simulink model "HilBlkFilterDemo"  (Simulink 6.0)
settings: Solver=FixedStepDiscrete  StartTime=0.0  StopTime=127/8000  RelTol=1e-3
StopFcn:
  | HilBlkFilterDemo_script('viewResults')
libraries: dspsrcs4 x2, HilLib x1, dsparch4 x1, dspsigops x1
settings Model: Creator=ckalluri  LastModifiedBy=mnazario
settings DataIOCC: SignalLoggingName=sigsOut
settings OptimizationCC: RollThreshold=2
settings DebuggingCC: CheckExecutionContextPreStartOutputMsg=on  CheckExecutionContextRuntimeOutputMsg=on  SolverPrmCheckMsg=none
settings HardwareCC: TargetUnknown=on
settings SFSimCC: SFSimApplyToAllLibs=on  SFSimBuildMode=Incremental

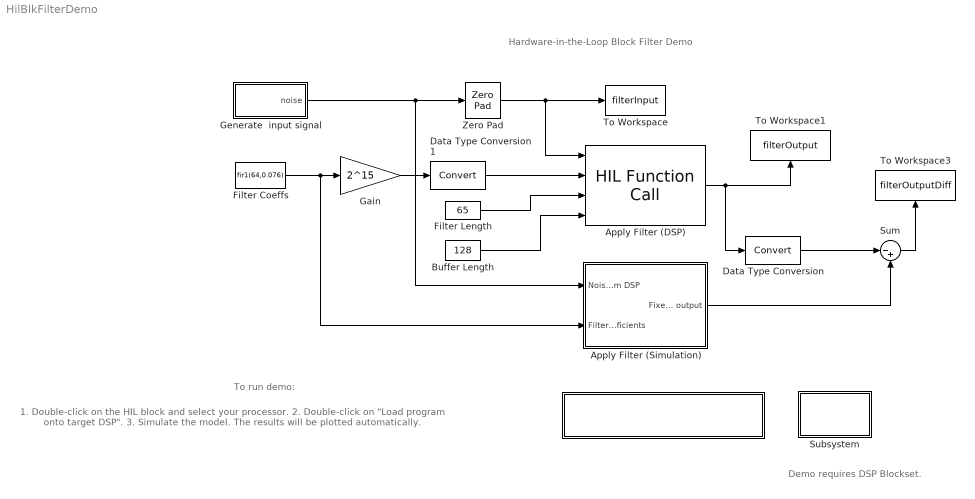
== system HilBlkFilterDemo ==
  note: Hardware-in-the-Loop Block
      | Filter Demo
  note: 1. Double-click on the HIL block and select your processor.
      | 2. Double-click on "Load program onto target DSP".
      | 3. Simulate the model.  The results will be plotted automatically.
  note: Demo requires DSP Blockset.
  note: To run demo:
  " " : Subsystem  PropExecContextAcrossSSBoundary=on
      settings: OpenFcn=HilBlkFilterDemo_script('loadProg')
      mask Display: disp('Load Program onto target DSP')
  Apply Filter (DSP) : HilLib/HIL Function Call
  Apply Filter (Simulation) : Subsystem  PropExecContextAcrossSSBoundary=on
      mask Display: disp('filter')
  Buffer Length : Constant  Value=128  OutDataTypeMode=uint16  SampleTime=128/8000
  Data Type Conversion : DataTypeConversion  OutDataTypeMode=double  SaturateOnIntegerOverflow=on  RndMeth=Zero
  Data Type Conversion1 : DataTypeConversion  OutDataTypeMode=int16  SaturateOnIntegerOverflow=on  RndMeth=Zero
  Filter Coeffs : Constant  Value=fir1(64,0.076)  OutDataTypeMode=double  SampleTime=128/8000
  Filter Length : Constant  Value=65  OutDataTypeMode=uint16  SampleTime=128/8000
  Gain : Gain  Gain=2^15  SaturateOnIntegerOverflow=on
  Generate  input signal : Subsystem  PropExecContextAcrossSSBoundary=on
  Subsystem : Subsystem  PropExecContextAcrossSSBoundary=on
      mask Display: disp('Info')
  Sum : Sum  Inputs=|-+  SaturateOnIntegerOverflow=on
  To Workspace : ToWorkspace  VariableName=filterInput  SampleTime=-1  SaveFormat=Array
  To Workspace1 : ToWorkspace  VariableName=filterOutput  SampleTime=-1  SaveFormat=Array
      settings: Orientation=up
  To Workspace3 : ToWorkspace  VariableName=filterOutputDiff  SampleTime=-1  SaveFormat=Array
      settings: Orientation=up
  Zero Pad : dspsigops/Zero Pad  padSigAt=Beginning  zpadAlong=Columns  padNumOutRowsSpecMethod=User-specified  numOutRows=128+65  padNumOutColsSpecMethod=User-specified  numOutCols=1  trunc_flag=None
  wires:
  Filter Length/1 -> Apply Filter (DSP)/3
  Buffer Length/1 -> Apply Filter (DSP)/4
  Apply Filter (Simulation)/1(Fixed-point output) -> Sum/2
  Data Type Conversion/1 -> Sum/1
  Sum/1 -> To Workspace3/1
  Filter Coeffs/1 -> Apply Filter (Simulation)/2(Filter Coefficients), Gain/1
  Data Type Conversion1/1 -> Apply Filter (DSP)/2
  Generate  input signal/1(noise) -> Apply Filter (Simulation)/1(Noisy Signal  from DSP), Zero Pad/1
  Gain/1 -> Data Type Conversion1/1
  Apply Filter (DSP)/1 -> Data Type Conversion/1, To Workspace1/1
  Zero Pad/1 -> To Workspace/1, Apply Filter (DSP)/1

== system HilBlkFilterDemo/  ==

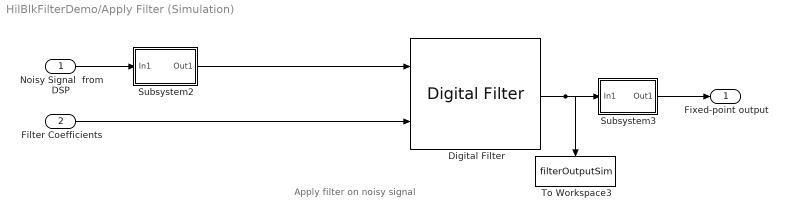
== system HilBlkFilterDemo/Apply Filter (Simulation) ==
  note: Apply filter on noisy signal
  Noisy Signal  from DSP : Inport  LatchInput=off
  Filter Coefficients : Inport  Port=2  LatchInput=off
  Digital Filter : dsparch4/Digital Filter  TypePopup=FIR (all zeros)  IIRFiltStruct=Direct form II transposed  AllPoleFiltStruct=Direct form  FIRFiltStruct=Direct form  CoeffSource=Input port(s)  NumCoeffs=[1 2]  DenCoeffs=[1 0.1]  BiQuadCoeffs=[1 0.3 0.4 1 0.1 0.2]  LatticeCoeffs=[0.2 0.4]  denIgnore=on  FiltPerSampPopup=One filter per frame  IC=0  ICnum=0  ICden=0  roundingMode=Floor  overflowMode=off
  Subsystem2 : Subsystem  PropExecContextAcrossSSBoundary=on
      mask Display: disp(sprintf('Scale'))
  Subsystem3 : Subsystem  PropExecContextAcrossSSBoundary=on
      mask Display: disp(sprintf('Scale'))
  To Workspace3 : ToWorkspace  VariableName=filterOutputSim  SampleTime=-1  SaveFormat=Array
      settings: Orientation=down
  Fixed-point output : Outport
  wires:
  Subsystem3/1(Out1) -> Fixed-point output/1
  Noisy Signal  from DSP/1 -> Subsystem2/1(In1)
  Subsystem2/1(Out1) -> Digital Filter/1
  Filter Coefficients/1 -> Digital Filter/2
  Digital Filter/1 -> Subsystem3/1(In1), To Workspace3/1

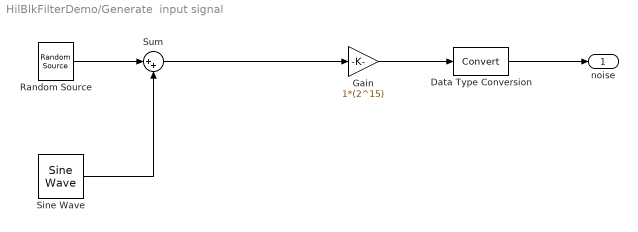
== system HilBlkFilterDemo/Generate  input signal ==
  Data Type Conversion : DataTypeConversion  OutDataTypeMode=int16  SaturateOnIntegerOverflow=on  RndMeth=Zero
  Gain : Gain  Gain=1*(2^15)  SaturateOnIntegerOverflow=on
  Random Source : dspsrcs4/Random Source  SrcType=Uniform  NormMethod=Ziggurat  CltLength=12  Min=-0.2  Max=0.2  Mean=0  Var=1  RepMode=Not repeatable  Seed=1  Inherit=off  SampMode=Discrete  SampTime=1/8000  SampFrame=128  DataType=Single  OutComplex=Real
  Sine Wave : dspsrcs4/Sine Wave  Amplitude=0.7  Frequency=200  Phase=0  SampleMode=Discrete  OutComplex=Real  CompMethod=Trigonometric fcn  TableSize=Speed  SampleTime=1/8000  SamplesPerFrame=128  dataType=single  wordLen=16  udDataType=sfix(16)  fracBitsMode=Best precision  numFracBits=15  ResetState=Restart at time zero
      settings: additionalParams=on
  Sum : Sum  Inputs=|++  SaturateOnIntegerOverflow=on  InputSameDT=on
  noise : Outport
  wires:
  Gain/1 -> Data Type Conversion/1
  Data Type Conversion/1 -> noise/1
  Sum/1 -> Gain/1
  Random Source/1 -> Sum/1
  Sine Wave/1 -> Sum/2

== system HilBlkFilterDemo/Subsystem ==
  note: This demo illustrates the use of the Hardware-In-The-Loop (HIL) block from Link for Code Composer Studio.
      | This block allows you to run individual functions on your target DSP, while using Simulink to provide inputs as well
      | as view and analyze the results of your implementation.
      |
      | The function being used is part of the 'filterFFT.pjt' project file in Code Composer Studio.
      |
      | The function is accessed via an HIL Function Call block. The inputs to the function are provided as Simulink inputs
      | to the HIL block.  The sizes of each of the arrays as well as the port direction (input or output) can be configured in the HIL block.
      | When configuring the sizes of these arrays, it is essential to ensure that these sizes are compatible with the other input parameters
      | to the function. For example, the filter input signal has length 193, so the HIL Block must be configured for a size of [193 1] on this input
      | port.
      |
      | To run the demo, you will first need to set up the appropriate processor in the HIL blocks. . In order to do this, double-click on the HIL block
      | and select the Target Selection tab. You can now select the Board name from the drop-down list to select the target where you want to
      | load and run the function.
      |
      | After setting up the HIL block to select the target, you will need to load the appropriate '.out' file. The demo comes with pre-built '.out' files
      | for the C67x/C62x, C64x, C54x, and C28x processor families.
      |
      | To load the program onto the target DSP, click on the 'Load Program onto Target DSP' button.
      |
      | Now run the demo by clicking Simulation => Start.  The results will be displayed automatically.

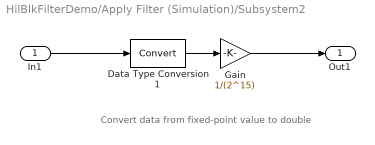
== system HilBlkFilterDemo/Apply Filter (Simulation)/Subsystem2 ==
  note: Convert data from fixed-point value to double
  In1 : Inport  LatchInput=off
  Data Type Conversion1 : DataTypeConversion  OutDataTypeMode=double  SaturateOnIntegerOverflow=on  RndMeth=Zero
  Gain : Gain  Gain=1/(2^15)  SaturateOnIntegerOverflow=on
  Out1 : Outport
  wires:
  Data Type Conversion1/1 -> Gain/1
  Gain/1 -> Out1/1
  In1/1 -> Data Type Conversion1/1

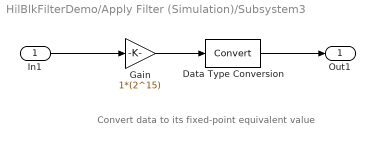
== system HilBlkFilterDemo/Apply Filter (Simulation)/Subsystem3 ==
  note: Convert data to its fixed-point equivalent value
  In1 : Inport  LatchInput=off
  Data Type Conversion : DataTypeConversion  OutDataTypeMode=double  SaturateOnIntegerOverflow=on  RndMeth=Zero
  Gain : Gain  Gain=1*(2^15)  SaturateOnIntegerOverflow=on
  Out1 : Outport
  wires:
  In1/1 -> Gain/1
  Gain/1 -> Data Type Conversion/1
  Data Type Conversion/1 -> Out1/1
